simulink model "labsys_heat"  (R2018b)
settings: Solver=ode15s  StartTime=0.0  StopTime=3600*7  FixedStep=1  RelTol=1e-3  AbsTol=1e-6
model workspace (MATLAB code in the model file):
  | % For MPC design to be used in LabSys
  | 
  | %disp('adding models...')
  | load('mpc_param_var05_opt_weight_du')
  | load('mpc_param_var05_uweight_01003')
  | load('mpc_param_var05_uweight_1')
  | load('tf8.mat')
  | 
  | 
  | %T_s=30;
  | %disp('done.')
undefined symbols (not defined in the file or in its folder): c, f, M, md, p, ref, refA, Req, T_s, timeUnit_1week, TinIC, Ts
libraries: instrumentlib x2, cstblocks x1, mpclib x1, simulink x1, dspnetwork x1, powerlib_meascontrol x1
Description:
  | Thermal Model of a House
  | 
  | This demo illustrates how you can use Simulink(R) to create the thermal model of
  | a house. This system models the outdoor environment, the thermal
  | characteristics of the house, and the house heating system.
  | 
  | The sldemo_househeat_data.m file initializes data in the model workspace.
  | To make changes, you can edit the model workspace directly or edit the MATLAB(R) file
  | and re-load the model workspace.
  | 
  | To view the model workspace, select View > Model Explorer
  | from the Simulink editor.
  | 
  | Note: Time is given in units of hours
settings Model: SimulationMode=accelerator  PauseTimes=3000  NumberOfSteps=600  ExtModeTrigMode=oneshot  ExtModeArmWhenConnect=off  ExtModeAutoUpdateStatusClock=off  Creator=The MathWorks, Inc.  LastModifiedBy=Gyulai László
settings SolverCC: AutoScaleAbsTol=off
settings DataIOCC: ExternalInput=[]  InitialState=[]  SaveFormat=StructureWithTime  SaveOutput=off  SaveTime=off  SignalLoggingName=sldemo_househeat_output
settings OptimizationCC: BlockReduction=off  BooleanDataType=off  ExpressionDepthLimit=2147483647  InitFltsAndDblsToZero=on  EfficientMapNaN2IntZero=off  LifeSpan=inf  BufferReusableBoundary=off
settings DebuggingCC: SaveWithParameterizedLinksMsg=none  UnderspecifiedInitializationDetection=Classic  MergeDetectMultiDrivingBlocksExec=none  SignalResolutionControl=TryResolveAllWithWarning  MultiTaskDSMMsg=warning  MultiTaskCondExecSysMsg=none  IntegerOverflowMsg=none  FcnCallInpInsideContextMsg=warning  BusObjectLabelMismatch=none  StateNameClashWarn=warning  SFUnexpectedBacktrackingDiag=warning  SFNoUnconditionalDefaultTransitionDiag=warning  SFExecutionAtInitializationDiag=none  IntegerSaturationMsg=none
settings HardwareCC: ProdBitPerPointer=32  ProdBitPerSizeT=32  ProdBitPerPtrDiffT=32  ProdLargestAtomicFloat=None  ProdIntDivRoundTo=Undefined  ProdEndianess=Unspecified  ProdWordSize=32  ProdHWDeviceType=32-bit Generic  TargetBitPerPointer=64  TargetBitPerSizeT=64  TargetBitPerPtrDiffT=64  TargetLongLongMode=on  TargetIntDivRoundTo=Zero  TargetEndianess=LittleEndian  TargetWordSize=64  TargetHWDeviceType=MATLAB Host  ProdEqTarget=off
settings ModelReferenceCC: PropagateSignalLabelsOutOfModel=off
settings SFSimCC: SimUseLocalCustomCode=off
settings CodeAppCC: MaxIdLength=128
settings GRTTargetCC: TargetLangStandard=C89/C90 (ANSI)  CombineOutputUpdateFcns=off  GRTInterface=on
settings ConfigComp: CovMetricSettings=dw  CovHtmlReporting=on  CovSaveCumulativeToWorkspaceVar=on  CovSaveSingleToWorkspaceVar=on  CovExternalEMLEnable=off
settings SimscapeCC: SimscapeNormalizeSystem=off

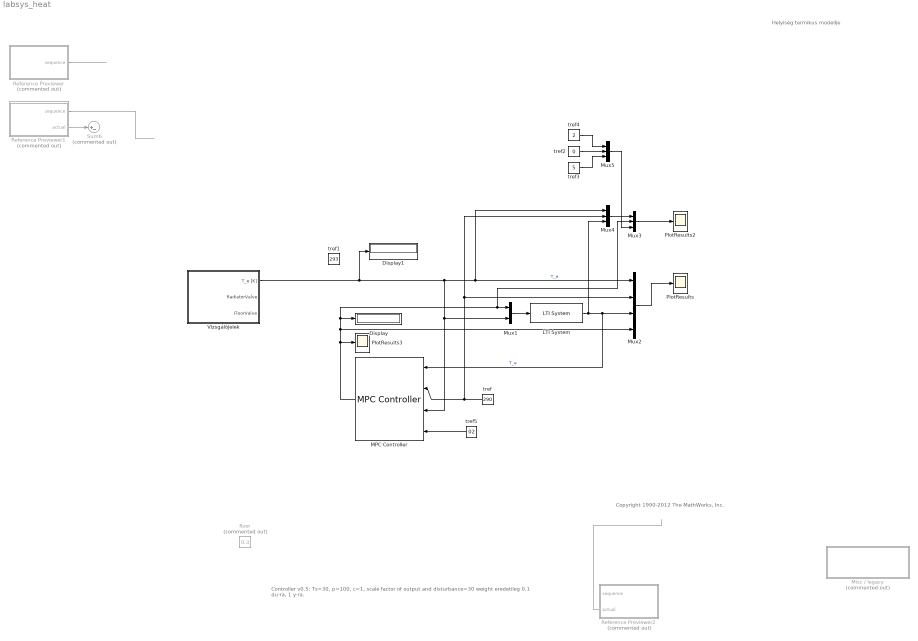
== system labsys_heat ==
  note: Controller v0.5: Ts=30, p=100, c=1, scale factor of output and disturbance=30
      | weight eredetileg 0.1 du-ra, 1 y-ra.
  note: Copyright 1990-2012 The MathWorks, Inc.
  note: Helyiség termikus modellje
  Display : Display
  Display1 : Display
  LTI System : cstblocks/LTI System  sys=tf8  IC=[]
  MPC Controller : mpclib/MPC Controller  SCDEnableBlockLinearizationSpecification=on  mpcobj=mpc_labsys05_u1  x0=mpcstate05  is_multiple=0  enable_value=0  return_u0=off  updateMPCinCallerWorkspace=on  md_inport=on  mv_inport=off  return_cost=off  return_mvseq=off  return_qpstatus=off  return_xseq=off  return_state=off  return_ovseq=off  state_inport=off  umin_inport=off  umax_inport=off  ymin_inport=off  ymax_inport=off  cc_inport=off  ywt_inport=off  uwt_inport=on  duwt_inport=off  rhoeps_inport=off  uref_inport=off  n_ts=30  n_p=100  n_mv=1  n_md=1  n_ud=0  n_mo=1  n_uo=0  BlockDataType=double  SampleTimeInherited=off  switch_inport=off
  Misc / legacy : Subsystem  Commented=on
  Mux1 : Mux  Inputs=2
  Mux2 : Mux
  Mux3 : Mux  Inputs=3
  Mux4 : Mux  Inputs=3
  Mux5 : Mux  Inputs=3
  PlotResults : Scope
  PlotResults2 : Scope
  PlotResults3 : Scope
  Reference Previewer : Subsystem  Commented=on  mask{signal=ref, ts=Ts, steps=p}
      mask prompts: signal "Signal name"; ts "Sampling time"; steps "Number of previewing steps"
      mask init:
      | ts = evalin('base',get_param(gcbh,'ts'));
      | signal = evalin('base',get_param(gcbh,'signal'));
      | steps = evalin('base',get_param(gcbh,'steps'));
      | data = mpc_previewer_maskinit(signal,ts);
      mask Display:
      | fprintf('Future\nsample\nextractor');
      | port_label('output', 1, 'seq')
      | port_label('output', 2, '@t')
  Reference Previewer1 : Subsystem  Commented=on  mask{signal=md, ts=Ts, steps=p}
      mask prompts: signal "Signal name"; ts "Sampling time"; steps "Number of previewing steps"
      mask init:
      | ts = evalin('base',get_param(gcbh,'ts'));
      | signal = evalin('base',get_param(gcbh,'signal'));
      | steps = evalin('base',get_param(gcbh,'steps'));
      | data = mpc_previewer_maskinit(signal,ts);
      mask Display:
      | fprintf('Future\nsample\nextractor');
      | port_label('output', 1, 'seq')
      | port_label('output', 2, '@t')
  Reference Previewer2 : Subsystem  Commented=on  mask{signal=refA, ts=Ts, steps=100}
      mask prompts: signal "Signal name"; ts "Sampling time"; steps "Number of previewing steps"
      mask init:
      | ts = evalin('base',get_param(gcbh,'ts'));
      | signal = evalin('base',get_param(gcbh,'signal'));
      | steps = evalin('base',get_param(gcbh,'steps'));
      | data = mpc_previewer_maskinit(signal,ts);
      mask Display:
      | fprintf('Future\nsample\nextractor');
      | port_label('output', 1, 'seq')
      | port_label('output', 2, '@t')
  Sum6 : Sum  Commented=on  Inputs=|+-  SaturateOnIntegerOverflow=on  InputSameDT=on  OutDataTypeStr=Inherit: Same as first input
  Vizsgálójelek : Subsystem
  floor : Constant  Commented=on  Value=0.3  SampleTime=300
  tref : Constant  Value=290  SampleTime=300
  tref1 : Constant  Value=293  SampleTime=300
  tref2 : Constant  Value=0  SampleTime=300
  tref3 : Constant  Value=5  SampleTime=300
  tref4 : Constant  Value=2  SampleTime=300
  tref5 : Constant  Value=02  SampleTime=300
  wires:
  Reference Previewer/1(sequence) -> ?
  Reference Previewer1/1(sequence) -> ?
  tref/1 -> Mux4/2, Mux2/2, MPC Controller/2
  Reference Previewer1/2(actual) -> Sum6/1
  Mux1/1 -> LTI System/1
  Mux2/1 -> PlotResults/1
  LTI System/1 -> Mux4/3, MPC Controller/1, Mux2/3  "T_e"
  Reference Previewer2/2(actual) -> ?
  Vizsgálójelek/1(T_e [K]) -> MPC Controller/3, Mux1/2, Mux4/1, Mux2/1, Display1/1  "T_e"
  Mux3/1 -> PlotResults2/1
  Mux4/1 -> Mux3/1
  MPC Controller/1 -> PlotResults3/1, Display/1, Mux3/2, Mux1/1, Mux2/4
  tref2/1 -> Mux5/2
  tref4/1 -> Mux5/1
  tref3/1 -> Mux5/3
  Mux5/1 -> Mux3/3
  tref5/1 -> MPC Controller/4

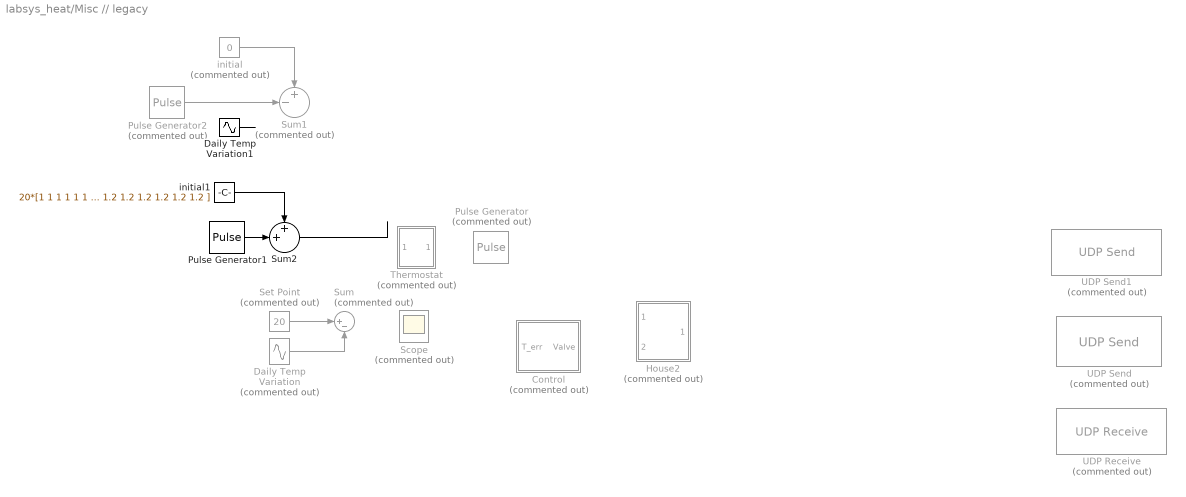
== system labsys_heat/Misc // legacy ==
  Control : Subsystem  Commented=on
  Daily Temp Variation : Sin  Commented=on  Amplitude=5  Frequency=3.14*2/3600/24  Phase=3.14/2  SampleTime=0
  Daily Temp Variation1 : Sin  Amplitude=5  Frequency=3.14*2/3600/24  Phase=3.14/2  SampleTime=300
  House2 : Subsystem  Commented=on
      mask Display: image(fullfile(matlabroot,'toolbox','simulink','simdemos','simgeneral','images','HouseHeatHousePix.svg'))
  Pulse Generator : DiscretePulseGenerator  Commented=on  PulseType=Time based  Period=3600*24*4  PulseWidth=50
  Pulse Generator1 : DiscretePulseGenerator  Amplitude=0  Period=12*24  PulseWidth=12  SampleTime=300
  Pulse Generator2 : DiscretePulseGenerator  Commented=on  Amplitude=0  Period=12*24  PulseWidth=12*4  SampleTime=300
  Scope : Scope  Commented=on
  Set Point : Constant  Commented=on  Value=20
  Sum : Sum  Commented=on  Inputs=+-|  SaturateOnIntegerOverflow=on  InputSameDT=on  OutDataTypeStr=Inherit: Same as first input
  Sum1 : Sum  Commented=on  Inputs=+-|  SaturateOnIntegerOverflow=on  InputSameDT=on  OutDataTypeStr=Inherit: Same as first input
  Sum2 : Sum  Inputs=++|  SaturateOnIntegerOverflow=on  InputSameDT=on  OutDataTypeStr=Inherit: Same as first input
  Thermostat : Subsystem  Commented=on
      mask Display: image(fullfile(matlabroot,'toolbox','simulink','simdemos','simgeneral','images','HouseHeatThermostatPix.svg'))
  UDP Receive : instrumentlib/UDP Receive  Commented=on  Host=localhost  Port=9090  LocalPort=-1  EnablePortSharing=off  GetLatestData=off  DataSize=[1 1]  DataType=uint8  ASCIIFormatting=%f,  Terminator=LF  ByteOrder=BigEndian  EnableBlockingMode=on  Timeout=10  SampleTime=0.01  LocalAddress=0.0.0.0
      settings: SourceProductName=Instrument Control Toolbox
  UDP Send : dspnetwork/UDP Send  Commented=on  remoteURL='127.0.0.1'  remotePort=25000  localURL='0.0.0.0'  localPortSource=Automatically determine  localPort=-1  sampletime=-1  blockPlatform=[]  separateLengthPort=0
      settings: SourceProductName=DSP System Toolbox  SourceProductBaseCode=DS
  UDP Send1 : instrumentlib/UDP Send  Commented=on  Port=9090  LocalPort=-1  EnablePortSharing=off  ByteOrder=BigEndian  OutputDatagramPacketSize=512  EnableBlockingMode=on  LocalAddress=0.0.0.0
      settings: SourceProductName=Instrument Control Toolbox
  initial : Constant  Commented=on  Value=0  SampleTime=300
  initial1 : Constant  Value=20*[1 1 1 1 1 1 1 1 1 1 1 1 1 1 1 1 1 1 1 1 1 1 1 1 1.2 1.2 1.2 1.2 1.2 1.2 1.2 1.2 1.2 1.2 1.2 1.2 1.2 1.2 1.2 1.2 1.2 1.2 1.2 1.2 1.2 1.2 1.2 1.2 ]  SampleTime=300
  wires:
  Set Point/1 -> Sum/1
  Daily Temp Variation/1 -> Sum/2
  Pulse Generator1/1 -> Sum2/2
  Pulse Generator2/1 -> Sum1/2
  initial1/1 -> Sum2/1
  Daily Temp Variation1/1 -> ?
  initial/1 -> Sum1/1
  Sum2/1 -> ?

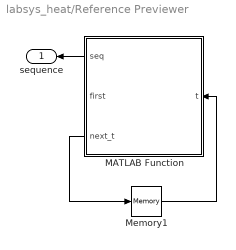
== system labsys_heat/Reference Previewer ==
  MATLAB Function : MATLAB Function  TreatAsAtomicUnit=on
  Memory1 : Memory  InheritSampleTime=on  LinearizeAsDelay=on
  sequence : Outport
  wires:
  MATLAB Function/1(seq) -> sequence/1
  Memory1/1 -> MATLAB Function/1(t)
  MATLAB Function/3(next_t) -> Memory1/1

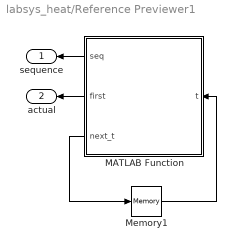
== system labsys_heat/Reference Previewer1 ==
  MATLAB Function : MATLAB Function  TreatAsAtomicUnit=on
  Memory1 : Memory  InheritSampleTime=on  LinearizeAsDelay=on
  sequence : Outport
  actual : Outport  Port=2
  wires:
  MATLAB Function/1(seq) -> sequence/1
  Memory1/1 -> MATLAB Function/1(t)
  MATLAB Function/3(next_t) -> Memory1/1
  MATLAB Function/2(first) -> actual/1

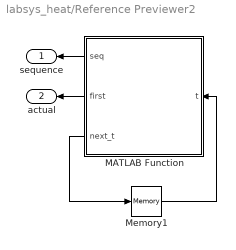
== system labsys_heat/Reference Previewer2 ==
  MATLAB Function : MATLAB Function  TreatAsAtomicUnit=on
  Memory1 : Memory  InheritSampleTime=on  LinearizeAsDelay=on
  sequence : Outport
  actual : Outport  Port=2
  wires:
  MATLAB Function/1(seq) -> sequence/1
  Memory1/1 -> MATLAB Function/1(t)
  MATLAB Function/3(next_t) -> Memory1/1
  MATLAB Function/2(first) -> actual/1

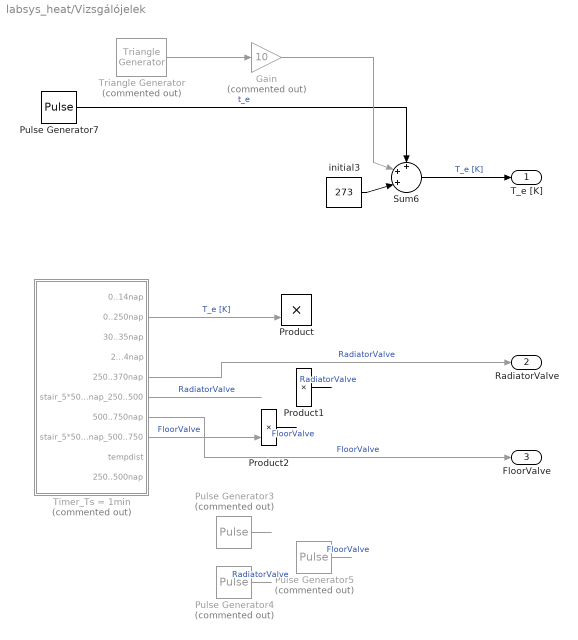
== system labsys_heat/Vizsgálójelek ==
  Gain : Gain  Commented=on  Gain=10
  Product : Product
  Product1 : Product
  Product2 : Product
  Pulse Generator3 : DiscretePulseGenerator  Commented=on  PulseType=Time based  Period=3600*24*30*3  PulseWidth=45  PhaseDelay=3600*24*20
  Pulse Generator4 : DiscretePulseGenerator  Commented=on  PulseType=Time based  Amplitude=0.5  Period=3600*24*30*3  PulseWidth=50
  Pulse Generator5 : DiscretePulseGenerator  Commented=on  PulseType=Time based  Period=3600*24*30*3  PulseWidth=40
  Pulse Generator7 : DiscretePulseGenerator  Amplitude=-2  Period=1800/30  PulseWidth=1800/60  SampleTime=30
  Sum6 : Sum  Inputs=+++|  SaturateOnIntegerOverflow=on  InputSameDT=on  OutDataTypeStr=Inherit: Same as first input
  Timer_Ts = 1min : Subsystem  Commented=on
  Triangle Generator : powerlib_meascontrol/Pulse & Signal Generators/Triangle Generator  Commented=on  Freq=1/(3600*12)  Phase=30  Ts=30
      settings: SourceProductName=Simscape Electrical
  initial3 : Constant  Value=273  SampleTime=1800
  T_e [K] : Outport
  RadiatorValve : Outport  Port=2
  FloorValve : Outport  Port=3
  wires:
  Product1/1 -> ?  "RadiatorValve"
  Timer_Ts = 1min/2(0..250nap) -> Product/2  "T_e [K]"
  initial3/1 -> Sum6/3
  Pulse Generator7/1 -> Sum6/1  "t_e"
  Timer_Ts = 1min/6(stair_5*50nap_250..500) -> ?  "RadiatorValve"
  ? -> Product2/1
  Triangle Generator/1 -> Gain/1
  ? -> Product1/1
  Timer_Ts = 1min/8(stair_5*50nap_500..750) -> Product2/2  "FloorValve"
  Sum6/1 -> T_e [K]/1  "T_e [K]"
  Timer_Ts = 1min/5(250..370nap) -> RadiatorValve/1  "RadiatorValve"
  Timer_Ts = 1min/7(500..750nap) -> FloorValve/1  "FloorValve"
  Pulse Generator5/1 -> ?  "FloorValve"
  ? -> Product1/2
  Pulse Generator3/1 -> ?
  Product2/1 -> ?  "FloorValve"
  Pulse Generator4/1 -> ?  "RadiatorValve"
  Gain/1 -> Sum6/2

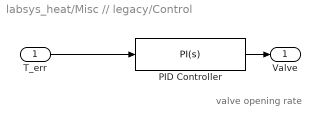
== system labsys_heat/Misc // legacy/Control ==
  note: valve opening rate
  T_err : Inport
  PID Controller : simulink/Continuous/PID Controller  Controller=PI  TimeDomain=Continuous-time  SampleTime=-1  IntegratorMethod=Forward Euler  FilterMethod=Forward Euler  Form=Parallel  UseFilter=on  ControllerParametersSource=internal  P=0.09  I=9.95e-07  D=0  N=100  InitialConditionSource=internal  InitialConditionForIntegrator=0  InitialConditionForFilter=0  ExternalReset=none  LimitOutput=on  UpperSaturationLimit=1  LowerSaturationLimit=0  LinearizeAsGain=on  AntiWindupMode=none  Kb=1  TrackingMode=off  Kt=1  PParamMin=[]  PParamMax=[]  IParamMin=[]  IParamMax=[]  DParamMin=[]  DParamMax=[]  NParamMin=[]  NParamMax=[]  KbParamMin=[]  KbParamMax=[]  KtParamMin=[]  KtParamMax=[]  POutMin=[]  POutMax=[]  IOutMin=[]  IOutMax=[]  DOutMin=[]  DOutMax=[]  NOutMin=[]  NOutMax=[]  KbOutMin=[]  KbOutMax=[]  KtOutMin=[]  KtOutMax=[]  IntegratorOutMin=[]  IntegratorOutMax=[]  FilterOutMin=[]  FilterOutMax=[]  SumOutMin=[]  SumOutMax=[]  SumI1OutMin=[]  SumI1OutMax=[]  SumI2OutMin=[]  SumI2OutMax=[]  SumI3OutMin=[]  SumI3OutMax=[]  SumDOutMin=[]  SumDOutMax=[]  SaturationOutMin=[]  SaturationOutMax=[]  IntegratorContinuousStateAttributes=''  IntegratorStateMustResolveToSignalObject=off  IntegratorRTWStateStorageClass=Auto  FilterContinuousStateAttributes=''  FilterStateMustResolveToSignalObject=off  FilterRTWStateStorageClass=Auto  DifferentiatorICPrevScaledInput=0  DifferentiatorOutMin=[]  DifferentiatorOutMax=[]
  Valve : Outport
  wires:
  T_err/1 -> PID Controller/1
  PID Controller/1 -> Valve/1

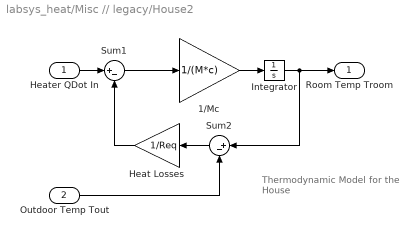
== system labsys_heat/Misc // legacy/House2 ==
  note: Thermodynamic Model
      | for the House
  Heater QDot In : Inport
  Outdoor Temp Tout : Inport  Port=2
  1/Mc : Gain  Gain=1/(M*c)  SaturateOnIntegerOverflow=on  OutDataTypeStr=Inherit: Same as input  ParamDataTypeStr=Inherit: Same as input
  Heat Losses : Gain  Gain=1/Req  SaturateOnIntegerOverflow=on  OutDataTypeStr=Inherit: Same as input  ParamDataTypeStr=Inherit: Same as input
  Integrator : Integrator  InitialCondition=TinIC
  Sum1 : Sum  Inputs=|+-  SaturateOnIntegerOverflow=on  InputSameDT=on  OutDataTypeStr=Inherit: Same as first input
  Sum2 : Sum  Inputs=|+-  SaturateOnIntegerOverflow=on  InputSameDT=on  OutDataTypeStr=Inherit: Same as first input
  Room Temp Troom : Outport  InitialOutput=0
  wires:
  Outdoor Temp Tout/1 -> Sum2/2
  Heater QDot In/1 -> Sum1/1
  Sum1/1 -> 1/Mc/1
  Sum2/1 -> Heat Losses/1
  Heat Losses/1 -> Sum1/2
  1/Mc/1 -> Integrator/1
  Integrator/1 -> Sum2/1, Room Temp Troom/1

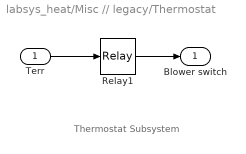
== system labsys_heat/Misc // legacy/Thermostat ==
  note: Thermostat Subsystem
  Terr : Inport
  Relay1 : Relay  OnSwitchValue=1  OffSwitchValue=-1
  Blower switch : Outport  InitialOutput=0
  wires:
  Terr/1 -> Relay1/1
  Relay1/1 -> Blower switch/1

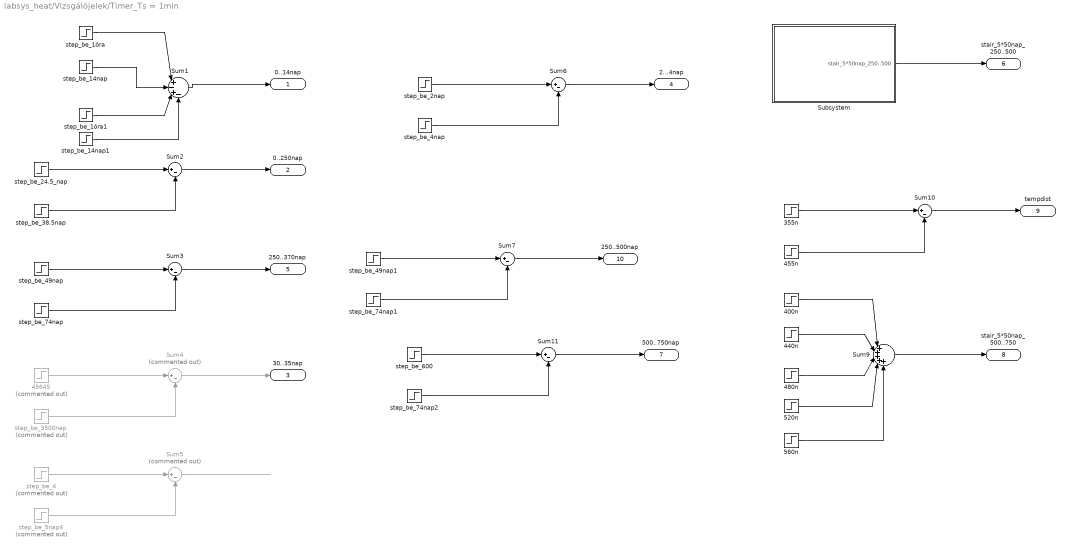
== system labsys_heat/Vizsgálójelek/Timer_Ts = 1min ==
  355n : Step  Time=3600*24*10*45  After=15  SampleTime=T_s
  400n : Step  Time=3600*24*10*50  After=0.1  SampleTime=T_s
  440n : Step  Time=3600*24*10*54  After=0.1  SampleTime=T_s
  455n : Step  Time=3600*24*10*50  After=20  SampleTime=T_s
  45645 : Step  Commented=on  Time=3600*24*30  SampleTime=0
  480n : Step  Time=3600*24*10*58  After=0.1  SampleTime=T_s
  520n : Step  Time=3600*24*10*62  After=0.3  SampleTime=T_s
  560n : Step  Time=3600*24*10*66  After=0.4  SampleTime=T_s
  Subsystem : Subsystem
  Sum1 : Sum  Inputs=|+-+-  SaturateOnIntegerOverflow=on  InputSameDT=on  OutDataTypeStr=Inherit: Same as first input
  Sum{2..3,6..7,10..11} (6 alike) : Sum  Inputs=|+-  SaturateOnIntegerOverflow=on  InputSameDT=on  OutDataTypeStr=Inherit: Same as first input
  Sum4 : Sum  Commented=on  Inputs=|+-  SaturateOnIntegerOverflow=on  InputSameDT=on  OutDataTypeStr=Inherit: Same as first input
  Sum5 : Sum  Commented=on  Inputs=|+-  SaturateOnIntegerOverflow=on  InputSameDT=on  OutDataTypeStr=Inherit: Same as first input
  Sum9 : Sum  Inputs=|+++++  SaturateOnIntegerOverflow=on  InputSameDT=on  OutDataTypeStr=Inherit: Same as first input
  step_be_14nap : Step  Time=timeUnit_1week*7*T_s  SampleTime=T_s
  step_be_14nap1 : Step  Time=timeUnit_1week*20*T_s  SampleTime=T_s
  step_be_1óra : Step  Time=0  SampleTime=T_s
  step_be_1óra1 : Step  Time=timeUnit_1week*17*T_s  SampleTime=T_s
  step_be_24.5_nap : Step  Time=0  SampleTime=T_s
  step_be_2nap : Step  Time=3600*24*2  SampleTime=0
  step_be_3500nap : Step  Commented=on  Time=3600*24*35  SampleTime=0
  step_be_38.5nap : Step  Time=3600*24*10*25  SampleTime=T_s
  step_be_4 : Step  Commented=on  Time=0  SampleTime=0
  step_be_49nap : Step  Time=3600*24*10*25  SampleTime=T_s
  step_be_49nap1 : Step  Time=3600*24*10*25  SampleTime=T_s
  step_be_4nap : Step  Time=3600*24*4  SampleTime=0
  step_be_5nap4 : Step  Commented=on  Time=3600*24*5  SampleTime=0
  step_be_600 : Step  Time=3600*24*10*50  SampleTime=T_s
  step_be_74nap : Step  Time=3600*24*10*45  SampleTime=T_s
  step_be_74nap1 : Step  Time=3600*24*10*50  SampleTime=T_s
  step_be_74nap2 : Step  Time=3600*24*10*70  SampleTime=T_s
  0..14nap : Outport
  0..250nap : Outport  Port=2
  30..35nap : Outport  Port=3
  2...4nap : Outport  Port=4
  250..370nap : Outport  Port=5
  stair_5*50nap_250..500 : Outport  Port=6
  500..750nap : Outport  Port=7
  stair_5*50nap_500..750 : Outport  Port=8
  tempdist : Outport  Port=9
  250..500nap : Outport  Port=10
  wires:
  Sum1/1 -> 0..14nap/1
  step_be_14nap/1 -> Sum1/2
  step_be_1óra/1 -> Sum1/1
  Sum2/1 -> 0..250nap/1
  step_be_38.5nap/1 -> Sum2/2
  step_be_24.5_nap/1 -> Sum2/1
  Sum3/1 -> 250..370nap/1
  step_be_74nap/1 -> Sum3/2
  step_be_49nap/1 -> Sum3/1
  Sum4/1 -> 30..35nap/1
  step_be_3500nap/1 -> Sum4/2
  45645/1 -> Sum4/1
  Sum5/1 -> ?
  step_be_5nap4/1 -> Sum5/2
  step_be_4/1 -> Sum5/1
  Sum6/1 -> 2...4nap/1
  step_be_4nap/1 -> Sum6/2
  step_be_2nap/1 -> Sum6/1
  step_be_14nap1/1 -> Sum1/4
  step_be_1óra1/1 -> Sum1/3
  Sum7/1 -> 250..500nap/1
  step_be_74nap1/1 -> Sum7/2
  step_be_49nap1/1 -> Sum7/1
  Sum9/1 -> stair_5*50nap_500..750/1
  440n/1 -> Sum9/2
  400n/1 -> Sum9/1
  520n/1 -> Sum9/4
  480n/1 -> Sum9/3
  560n/1 -> Sum9/5
  Sum10/1 -> tempdist/1
  455n/1 -> Sum10/2
  355n/1 -> Sum10/1
  Sum11/1 -> 500..750nap/1
  step_be_74nap2/1 -> Sum11/2
  step_be_600/1 -> Sum11/1
  Subsystem/1(stair_5*50nap_250..500) -> stair_5*50nap_250..500/1

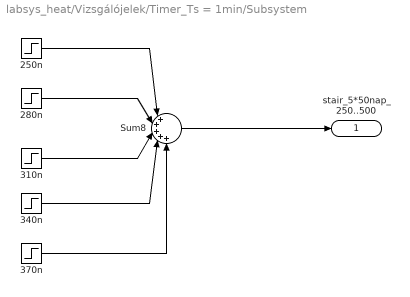
== system labsys_heat/Vizsgálójelek/Timer_Ts = 1min/Subsystem ==
  250n : Step  Time=3600*24*10*25  After=0.1  SampleTime=T_s
  280n : Step  Time=3600*24*10*29  After=0.1  SampleTime=T_s
  310n : Step  Time=3600*24*10*33  After=0.2  SampleTime=T_s
  340n : Step  Time=3600*24*10*37  After=0.2  SampleTime=T_s
  370n : Step  Time=3600*24*10*41  After=0.4  SampleTime=T_s
  Sum8 : Sum  Inputs=|+++++  SaturateOnIntegerOverflow=on  InputSameDT=on  OutDataTypeStr=Inherit: Same as first input
  stair_5*50nap_250..500 : Outport
  wires:
  370n/1 -> Sum8/5
  280n/1 -> Sum8/2
  340n/1 -> Sum8/4
  310n/1 -> Sum8/3
  250n/1 -> Sum8/1
  Sum8/1 -> stair_5*50nap_250..500/1

== matlab function labsys_heat/Reference Previewer/MATLAB Function ==
  settings: updateMethod=DISCRETE  sampleTime=ts
  data: data parameter double; seq output double; steps parameter double; t input double; first output double; next_t output double
function [seq,first,next_t] = fcn(data,steps,t)
%#codegen
[seq,first,next_t] = mpcblock_preview('ref',data,steps,t);

== matlab function labsys_heat/Reference Previewer1/MATLAB Function ==
  settings: updateMethod=DISCRETE  sampleTime=ts
  data: data parameter double; seq output double; steps parameter double; t input double; first output double; next_t output double
function [seq,first,next_t] = fcn(data,steps,t)
%#codegen
[seq,first,next_t] = mpcblock_preview('ref',data,steps,t);

== matlab function labsys_heat/Reference Previewer2/MATLAB Function ==
  settings: updateMethod=DISCRETE  sampleTime=ts
  data: data parameter double; seq output double; steps parameter double; t input double; first output double; next_t output double
function [seq,first,next_t] = fcn(data,steps,t)
%#codegen
[seq,first,next_t] = mpcblock_preview('ref',data,steps,t);
